simulink model "cdma2000_phlayer"  (Simulink 6.0)
settings: Solver=FixedStepDiscrete  SolverMode=SingleTasking  StartTime=0.0  StopTime=1  RelTol=1e-3
PreLoadFcn:
  | % Create interleaver table
  | % By default, numSampInt is set to 768 and radConfig to 3
  | interTable = cdma2000_inttable(768, 3);
undefined symbols (not defined in the file or in its folder): figposition, Fs, Non, slcm, TD
libraries: cdma2000_lib x8, commsink2 x5, commsequence2 x3, dspsigops x3, dspsnks4 x2, commblkintrlv2 x2, commcrc2 x2, commcnvcod2 x2, commrandsrc2 x1, commutil2 x1, dspsrcs4 x1
CloseFcn:
  | % Clear interleaver Table
  | clear interTable;
  | % Clear error string
  | clear eStr;
  | % Clear signal logging
  | clear cdma2000SigsOut;
settings Model: Creator=arodrigu  LastModifiedBy=arodrigu  ProdHWDeviceType=Specified
settings DataIOCC: LimitDataPoints=off  SaveOutput=off  SaveTime=off  SignalLoggingName=cdma2000SigsOut
settings OptimizationCC: BooleanDataType=off  InlineInvariantSignals=off
settings DebuggingCC: CheckExecutionContextPreStartOutputMsg=on  CheckExecutionContextRuntimeOutputMsg=on  SolverPrmCheckMsg=none  InheritedTsInSrcMsg=none
settings HardwareCC: ProdHWDeviceType=Specified
settings ModelReferenceCC: UpdateModelReferenceTargets=IfOutOfDate
settings CodeAppCC: MangleLength=5

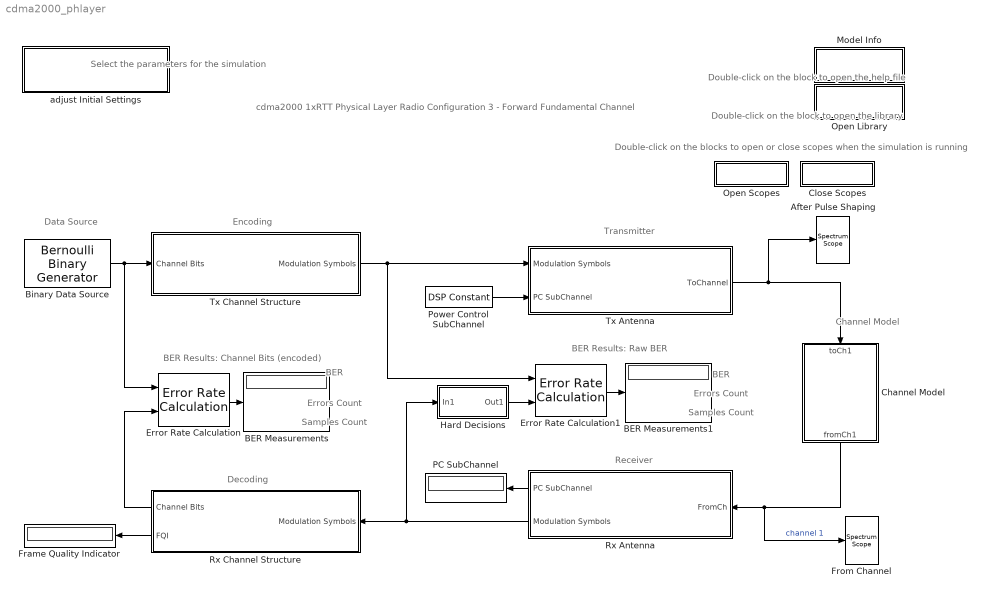
== system cdma2000_phlayer ==
  note: cdma2000 1xRTT Physical Layer
      | Radio Configuration 3 - Forward Fundamental Channel
  note: Double-click on the block
      | to open the help file
  note: BER
  note: Errors Count
  note: Samples Count
  note: BER
  note: Errors Count
  note: Samples Count
  note: Transmitter
  note: Receiver
  note: Channel
      | Model
  note: Encoding
  note: Decoding
  note: Select the parameters
      | for the simulation
  note: BER Results: Raw BER
  note: BER Results: Channel Bits (encoded)
  note: Double-click on the block
      | to open the library
  note: Double-click on the blocks to open or close scopes
      | when the simulation is running
  note: Data Source
  After Pulse Shaping : dspsnks4/Spectrum Scope  ScopeProperties=off  Domain=Frequency  HorizSpan=1  UseBuffer=on  BufferSize=256  Overlap=0  inpFftLenInherit=off  FFTlength=128  numAvg=20  DisplayProperties=on  AxisGrid=on  Memory=off  FrameNumber=off  AxisLegend=off  AxisZoom=off  OpenScopeAtSimStart=off  OpenScopeImmediately=off  FigPos="figposition([7    12    39    27])"  AxisProperties=off  XUnits=Hertz  XRange=[-Fs/2...Fs/2]  InheritXIncr=on  XIncr=1.0  XLabel=Samples  YUnits=dB  YLabel=Magnitude, dB  LineProperties=off  LineColors=[1 0 0]
      settings: YMin=-50.9192306956859  YMax=14.9570095672604
  BER Measurements : Display
  BER Measurements1 : Display
  Binary Data Source : commrandsrc2/Bernoulli Binary Generator  P=0.5  seed=1234  Ts=20e-3*1/172  frameBased=on  sampPerFrame=172  orient=off
      settings: AttributesFormatString=Samples per Frame = %<sampPerFrame>\nSample Time = %<Ts>
  Channel Model : Subsystem  Orientation=down  PropExecContextAcrossSSBoundary=on
      mask Display: disp('Channel\nModels');
  Close Scopes : Subsystem  PropExecContextAcrossSSBoundary=on
      settings: OpenFcn=|
      | str1 = 'Rx Antenna';
      | str2 = 'From Channel';
      | str3 = 'After Rake';
      | str5 = 'After Derotation';                                        str6 = 'After Pulse Shaping';
      | str7 = 'From Channel';
      | 
      | 
      | sdspfscope2([],[],[],'ScopeUpdate',[bdroot '/' str1 '/' str2 ],'CloseFig');
      | sdspfscope2([],[],[],'ScopeUpdate',[bdroot '/' str1 '/' str3 ],'CloseFig');
      | sdspfscope2([],[],[],'ScopeUpdate',[bdroot '/' str1 '/' str5 ],'CloseFig');
      | sdspfscope2([],[],[],'ScopeUpdate',[bdroot '/' str6],'CloseFig');
      |  sdspfscope2([],[],[],'ScopeUpdate',[bdroot '/' str7],'CloseFig');
      mask Display: disp('Close Scopes');
  Error Rate Calculation : commsink2/Error Rate Calculation  N=2*172  st_delay=0  cp_mode=Entire frame  subframe=[]  PMode=Port  WsName=ErrorVec  RsMode2=off  stop=off  numErr=100  maxBits=1e6
      settings: AttributesFormatString=Received Delay = %<N>
  Error Rate Calculation1 : commsink2/Error Rate Calculation  N=2*768  st_delay=0  cp_mode=Entire frame  subframe=[]  PMode=Port  WsName=ErrorVec  RsMode2=off  stop=off  numErr=100  maxBits=1e6
      settings: AttributesFormatString=Received Delay = %<N>
  Frame Quality Indicator : Display
  From Channel : dspsnks4/Spectrum Scope  ScopeProperties=off  Domain=Frequency  HorizSpan=1  UseBuffer=on  BufferSize=512  Overlap=0  inpFftLenInherit=off  FFTlength=128  numAvg=2  DisplayProperties=on  AxisGrid=on  Memory=off  FrameNumber=off  AxisLegend=off  AxisZoom=off  OpenScopeAtSimStart=off  OpenScopeImmediately=off  FigPos="figposition([49    12    39    27])"  AxisProperties=off  XUnits=Hertz  XRange=[-Fs/2...Fs/2]  InheritXIncr=on  XIncr=1.0  XLabel=Samples  YUnits=dB  YLabel=Magnitude, dB  LineProperties=off  LineColors=[1 0 0]
      settings: YMin=-25.3833693734741  YMax=21.0980719822277
  Hard Decisions : Subsystem  PropExecContextAcrossSSBoundary=on
      mask Display: disp('Hard\nDecisions');
  Model Info : Subsystem  LoadFcn=slcm LoadBlock;  InitFcn=slcm('UpdateAllCMBlocksInThisModelInit')  PropExecContextAcrossSSBoundary=on  mask(CMBlock){InitialSaveTempField=, InitialBlockCM=None, BlockCM=None, Frame=on, SaveTempField=, DisplayStringWithTags=Info, MaskDisplayString=Info, HorizontalTextAlignment=Center, LeftAlignmentValue=0.5, SourceBlockDiagram=cdma2000_phlayer, TagMaxNumber=20, CMTag1=, CMTag2=, CMTag3=, CMTag4=, CMTag5=, CMTag6=, CMTag7=, CMTag8=, CMTag9=, CMTag10=, CMTag11=, CMTag12=, CMTag13=, CMTag14=, CMTag15=, CMTag16=, CMTag17=, CMTag18=, CMTag19=, CMTag20=}
      mask help: This block allows revision control information to be displayed within the model.
      settings: CopyFcn=slcm CopyBlock;  DeleteFcn=slcm Cancel;  PostSaveFcn=slcm('UpdateAllCMBlocksInThisModel')  NameChangeFcn=slcm Rename;  OpenFcn=commdemohelp;
      mask Display: text(str2num(LeftAlignmentValue), 0.5, MaskDisplayString, 'HorizontalAlignment', HorizontalTextAlignment)
  Open Library : Subsystem  PropExecContextAcrossSSBoundary=on
      settings: OpenFcn=open('cdma2000_lib.mdl');
      mask Display: disp('cdma2000\nLibrary')
  Open Scopes : Subsystem  PropExecContextAcrossSSBoundary=on
      settings: OpenFcn=|
      | str1 = 'Rx Antenna';
      | str2 = 'From Channel';
      | str3 = 'After Rake';
      | str5 = 'After Derotation';
      | str6 = 'After Pulse Shaping';
      | str7 = 'From Channel';
      | 
      | sdspfscope2([],[],[],'ScopeUpdate',[bdroot '/' str1 '/' str2 ],'OpenFig');
      | sdspfscope2([],[],[],'ScopeUpdate',[bdroot '/' str1 '/' str3 ],'OpenFig');
      | sdspfscope2([],[],[],'ScopeUpdate',[bdroot '/' str1 '/' str5 ],'OpenFig');
      | sdspfscope2([],[],[],'ScopeUpdate',[bdroot '/' str6],'OpenFig');
      |  sdspfscope2([],[],[],'ScopeUpdate',[bdroot '/' str7],'OpenFig');
      mask Display: disp('Open Scopes');
  PC SubChannel : Display
  Power Control SubChannel : dspsrcs4/DSP Constant  Value=1  SampleMode=Discrete  discreteOutput=Frame-based  continuousOutput=Sample-based  sampTime=20e-3/16  framePeriod=20e-3/16  dataType=Inherit from 'Constant value'  isSigned=on  wordLen=16  udDataType=sfix(16)  fracBitsMode=Best precision  numFracBits=15  InterpretAs1D=off  Ts=20e-3/16  FramebasedOutput=on
      settings: AttributesFormatString=\n\n\n\n
  Rx Antenna : Subsystem  Orientation=left  PropExecContextAcrossSSBoundary=on
  Rx Channel Structure : Subsystem  Orientation=left  PropExecContextAcrossSSBoundary=on
  Tx Antenna : Subsystem  PropExecContextAcrossSSBoundary=on
  Tx Channel Structure : Subsystem  PropExecContextAcrossSSBoundary=on
      mask Display:
      | port_label('output',1,'Modulation Symbols');
      | port_label('input',1,'Channel Bits');
  adjust Initial Settings : Subsystem  PropExecContextAcrossSSBoundary=on  mask(cdma2000 Initial Settings){chType=Forward Fundamental, radConfig=Radio Configuration 3, dataRates=9.6 Kbps, nFrameMask=1, longCScrMask=On, gateRateMask=1/4, trChCode=23, pnOffset=1, qof_idx=2, TxDivMode=Non-TD, chMode1=Multipath Fading Channel, EcN0=10, dopplerFreq=486, delayVector=[0 260e-9 521e-9 781e-9], gainVector=[0 -3 -6 -9]}
      mask prompts: chType "Channel Type"; radConfig "Radio Configuration"; dataRates "Data Rates:"; nFrameMask "Length of frame in multiples of 20 ms (n):"; longCScrMask "Long Code Scrambling:"; gateRateMask "Power Control SubChannel Insertion Rate:"; trChCode "Forward Traffic Channel Spreading Code Index:"; pnOffset "Forward Traffic Channel PN Offset:"; qof_idx "Quasi-orthogonal function index for F-DTCH:"; TxDivMode "Transmit Diversity Mode:"; chMode1 "Channel Model:"; EcN0 "EcN0 (in dB):"; dopplerFreq "Maximum Doppler Frequency shift (in Hz):"; delayVector "Multipath Profile - Delay Vector (s):"; gainVector "Multipath Profile - Gain Vector (dB):"
      mask help:
      | Select the parameters for the cdma200 application example.
      |
      | Some options have been disabled because they are not supported in this example. These options are intentionally displayed to exemplify possible ways to expand the model.
      mask init:
      | eStr = cdma2000_initmask(gcb, 'init');
      | if(~isempty(eStr.emsg))
      | errordlg(eStr.emsg);
      | end
      settings: AttributesFormatString=%<chType>\n%<radConfig>\n%<dataRates>\n%<txDivMode>\n%<chMode1>\n
      mask Help: eval('commdemohelp;');
      mask StyleString: popup(Forward Fundamental),popup(Radio Configuration 3),popup(1.5 Kbps|2.7 Kbps|4.8 Kbps|9.6 Kbps),popup(1|2|4),popup(On|Off),popup(Non Power Control|1|1/2|1/4),edit,edit,popup(0|1|2|3),popup(Non-TD),popup(No Channel|AWGN Channel|Multipath Fading Channel),edit,edit,edit,edit
      mask CallbackString: ||cdma2000_initmask(gcb,'cbDataRates');|cdma2000_initmask(gcb,'cbNFrameMask');|cdma2000_initmask(gcb,'cbLongCScrMask');|cdma2000_initmask(gcb,'cbGateRateMask');|cdma2000_initmask(gcb,'cbTrChCode');|cdma2000_initmask(gcb,'cbPnOffset');|cdma2000_initmask(gcb,'cbQof_idx');|cdma2000_initmask(gcb,'cbTxDivMode');|cdma2000_initmask(gcb,'cbChMode1');||||
      mask Display: disp('cdma2000:\nInitial Settings');
  wires:
  Binary Data Source/1 -> Tx Channel Structure/1(Channel Bits), Error Rate Calculation/1
  Error Rate Calculation/1 -> BER Measurements/1
  Error Rate Calculation1/1 -> BER Measurements1/1
  Tx Antenna/1(ToChannel) -> Channel Model/1(toCh1), After Pulse Shaping/1
  Channel Model/1(fromCh1) -> Rx Antenna/1(FromCh), From Channel/1  "channel 1"
  Tx Channel Structure/1(Modulation Symbols) -> Error Rate Calculation1/1, Tx Antenna/1(Modulation Symbols)
  Rx Channel Structure/1(Channel Bits) -> Error Rate Calculation/2
  Rx Channel Structure/2(FQI) -> Frame Quality Indicator/1
  Power Control SubChannel/1 -> Tx Antenna/2(PC SubChannel)
  Rx Antenna/1(PC SubChannel) -> PC SubChannel/1
  Rx Antenna/2(Modulation Symbols) -> Rx Channel Structure/1(Modulation Symbols), Hard Decisions/1(In1)
  Hard Decisions/1(Out1) -> Error Rate Calculation1/2

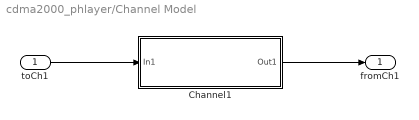
== system cdma2000_phlayer/Channel Model ==
  toCh1 : Inport  LatchInput=off
  Channel1 : Subsystem  BlockChoice=Multipath Fading Channel  PropExecContextAcrossSSBoundary=on
      link override AWGN Channel: EsNodB=10
      link override Multipath Fading Channel: EcN0=10  dopplerFreq=486  delayVector="[0    2.6e-007   5.21e-007   7.81e-007]"  gainVector=[0 -3 -6 -9]
      link override Multipath Fading Channel/AWGN Channel: EsNodB=EcN0
      link override Multipath Fading Channel/Multipath Rayleigh Fading Channel: Fd=dopplerFreq  delayVec=delayVector  gainVecdB=gainVector
      settings: AttributesFormatString=%<BlockChoice>  MemberBlocks=AWGN Channel,Multipath Fading Channel,No Channel
      settings: TemplateBlock=|
      | cdma2000_lib/cdma2000 Channel Models/Configurable
      | Subsystem
  fromCh1 : Outport
  wires:
  toCh1/1 -> Channel1/1(In1)
  Channel1/1(Out1) -> fromCh1/1

== system cdma2000_phlayer/Close Scopes ==
  note: This subsystem is intentionally left empty

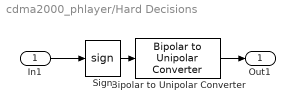
== system cdma2000_phlayer/Hard Decisions ==
  In1 : Inport  LatchInput=off
  Bipolar to Unipolar Converter : commutil2/Bipolar to Unipolar Converter  M=2  polarity=Negative
  Sign : Signum
  Out1 : Outport
  wires:
  Sign/1 -> Bipolar to Unipolar Converter/1
  Bipolar to Unipolar Converter/1 -> Out1/1
  In1/1 -> Sign/1

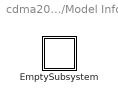
== system cdma2000_phlayer/Model Info ==
  EmptySubsystem : Subsystem  PropExecContextAcrossSSBoundary=on

== system cdma2000_phlayer/Open Library ==
  note: This subsystem is intentionally left empty

== system cdma2000_phlayer/Open Scopes ==
  note: This subsystem is intentionally left empty

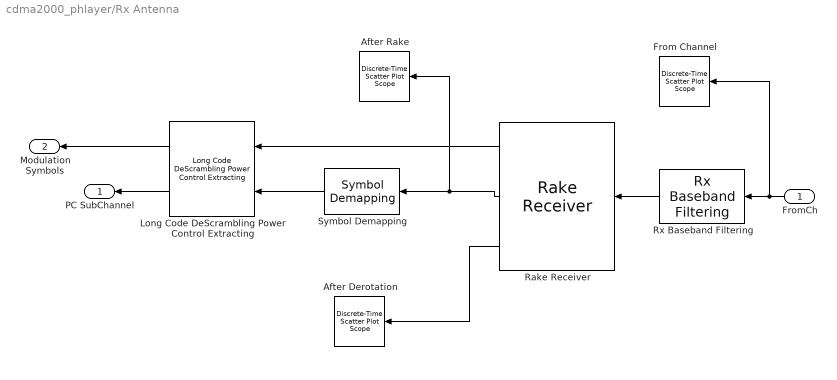
== system cdma2000_phlayer/Rx Antenna ==
  FromCh : Inport  Orientation=left  LatchInput=off
  After Derotation : commsink2/Discrete-Time Scatter Plot Scope  Tag=ScatterPlot  Orientation=left  sampPerSymb=1  offsetEye=0  numTraces=100  numNewFrames=20  LineMarkers=.  LineColors=b  fading=on  render=off  AxisGrid=on  xMin=-3.22434444007457  xMax=3.46614847196624  yMin=-3.31792338934159  yMax=3.37256952269922  inphaseLabel=After Derotation  quadratureLabel=""  openScopeAtSimStart=off  FrameNumber=off  FigPos="figposition([36    51    30    40])"  figTitle=.  numLinesMax=50  block_type_=scatter
  After Rake : commsink2/Discrete-Time Scatter Plot Scope  Tag=ScatterPlot  Orientation=left  sampPerSymb=1  offsetEye=0  numTraces=100  numNewFrames=40  LineMarkers=.  LineColors=[1 0 1]  fading=on  render=off  AxisGrid=on  xMin=-2.7  xMax=2.7  yMin=-2.7  yMax=2.7  inphaseLabel=After Rake Receiver  quadratureLabel=""  openScopeAtSimStart=off  FrameNumber=off  FigPos="figposition([68    51    30    40])"  figTitle=.  numLinesMax=50  block_type_=scatter
  From Channel : commsink2/Discrete-Time Scatter Plot Scope  Tag=ScatterPlot  Orientation=left  sampPerSymb=1  offsetEye=0  numTraces=3000  numNewFrames=2000  LineMarkers=.  LineColors=[1 0 1]  fading=on  render=off  AxisGrid=on  xMin=-2.7  xMax=2.7  yMin=-2.7  yMax=2.7  inphaseLabel=From Channel  quadratureLabel=""  openScopeAtSimStart=off  FrameNumber=off  FigPos="figposition([4    51    30    40])"  figTitle=.  numLinesMax=50  block_type_=scatter
  Long Code DeScrambling Power Control Extracting : cdma2000_lib/cdma2000 Receiver/Long Code DeScrambling Power Control Extracting  Orientation=left  radConfig=Radio Configuration 3  numSamp=768  nFrameMask=1  longCScrMask=On  gateRateMask=1/4  TxDivMode=Non-TD  plcMask="[1 1 0 0 0 1  1  0  0  1  1  0  1  0  1  1  1  1  0  1  1  0  0  1  0  1  1  1  0  0  1  0  1  0  1  1  1  1  0  1  1  0]"
  Rake Receiver : cdma2000_lib/cdma2000 Receiver/Rake Receiver  Orientation=left  walshLength=64  trChCode=23  pnOffset=1  qof_idx=2  numTapsChEst=11  numTapsRRC=48  overSampling=4  fingerEnables="[1  1  1  1]"  fingerPhases="[0  1  3  4]"
  Rx Baseband Filtering : cdma2000_lib/cdma2000 Receiver/Rx Baseband Filtering  Orientation=left
  Symbol Demapping : cdma2000_lib/cdma2000 Receiver/Symbol Demapping  Orientation=left
  PC SubChannel : Outport  Orientation=left
  Modulation Symbols : Outport  Orientation=left  Port=2
  wires:
  Rake Receiver/2 -> Symbol Demapping/1, After Rake/1
  Rake Receiver/1 -> Long Code DeScrambling Power Control Extracting/1
  Rx Baseband Filtering/1 -> Rake Receiver/1
  Long Code DeScrambling Power Control Extracting/1 -> Modulation Symbols/1
  FromCh/1 -> Rx Baseband Filtering/1, From Channel/1
  Long Code DeScrambling Power Control Extracting/2 -> PC SubChannel/1
  Rake Receiver/3 -> After Derotation/1
  Symbol Demapping/1 -> Long Code DeScrambling Power Control Extracting/2

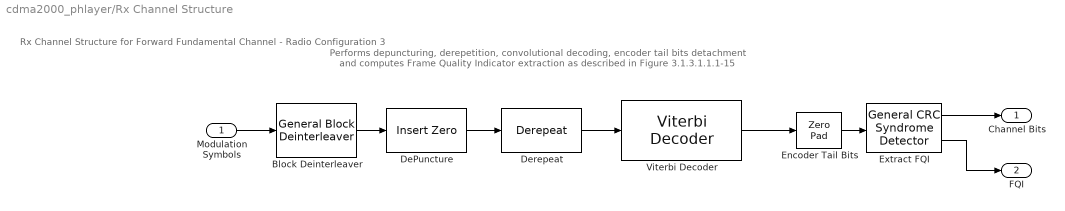
== system cdma2000_phlayer/Rx Channel Structure ==
  note: Rx Channel Structure for
      | Forward Fundamental Channel - Radio Configuration 3
  note: Performs depuncturing, derepetition, convolutional decoding, encoder tail bits detachment and computes
      | Frame Quality Indicator extraction as described in Figure 3.1.3.1.1.1-15
  Modulation Symbols : Inport  LatchInput=off
  Block Deinterleaver : commblkintrlv2/General Block Deinterleaver  elements=interTable
  DePuncture : commsequence2/Insert Zero  insertZeroVector=[1]
  Derepeat : commsequence2/Derepeat  N=1  ic=0  mode=Maintain input frame rate
  Encoder Tail Bits : dspsigops/Zero Pad  padSigAt=End  zpadAlong=Columns  padNumOutRowsSpecMethod=User-specified  numOutRows=172 + 12  padNumOutColsSpecMethod=User-specified  numOutCols=1  trunc_flag=None
  Extract FQI : commcrc2/General CRC Syndrome Detector  genPoly=[12 11 10 9 8 4 1 0]  iniStates=[1]  numChecksums=1
  Viterbi Decoder : commcnvcod2/Viterbi Decoder  trellis=poly2trellis(9, [765 671 513 473])  dectype=Unquantized  nsdecb=4  tbdepth=30  opmode=Truncated  reset=off
  Channel Bits : Outport
  FQI : Outport  Port=2
  wires:
  Block Deinterleaver/1 -> DePuncture/1
  Extract FQI/1 -> Channel Bits/1
  Extract FQI/2 -> FQI/1
  Encoder Tail Bits/1 -> Extract FQI/1
  Modulation Symbols/1 -> Block Deinterleaver/1
  Viterbi Decoder/1 -> Encoder Tail Bits/1
  Derepeat/1 -> Viterbi Decoder/1
  DePuncture/1 -> Derepeat/1

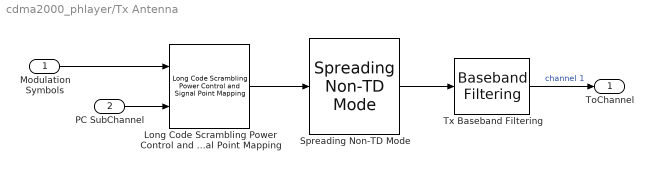
== system cdma2000_phlayer/Tx Antenna ==
  Modulation Symbols : Inport  LatchInput=off
  PC SubChannel : Inport  Port=2  LatchInput=off
  Long Code Scrambling Power Control and Signal Point Mapping : cdma2000_lib/cdma2000 Transmitter/Long Code Scrambling Power Control and Signal Point Mapping  radConfig=Radio Configuration 3  numSamp=768  nFrameMask=1  longCScrMask=On  gateRateMask=1/4  TxDivMode=Non-TD  plcMask="[1 1 0 0 0 1  1  0  0  1  1  0  1  0  1  1  1  1  0  1  1  0  0  1  0  1  1  1  0  0  1  0  1  0  1  1  1  1  0  1  1  0]"
  Spreading Non-TD Mode : cdma2000_lib/cdma2000 Transmitter/Spreading Non-TD Mode  walshLength=64  trChCode=23  qof_idx=2  pnOffset=1
  Tx Baseband Filtering : cdma2000_lib/cdma2000 Transmitter/Baseband Filtering
  ToChannel : Outport
  wires:
  PC SubChannel/1 -> Long Code Scrambling Power Control and Signal Point Mapping/2
  Long Code Scrambling Power Control and Signal Point Mapping/1 -> Spreading Non-TD Mode/1
  Spreading Non-TD Mode/1 -> Tx Baseband Filtering/1
  Modulation Symbols/1 -> Long Code Scrambling Power Control and Signal Point Mapping/1
  Tx Baseband Filtering/1 -> ToChannel/1  "channel 1"

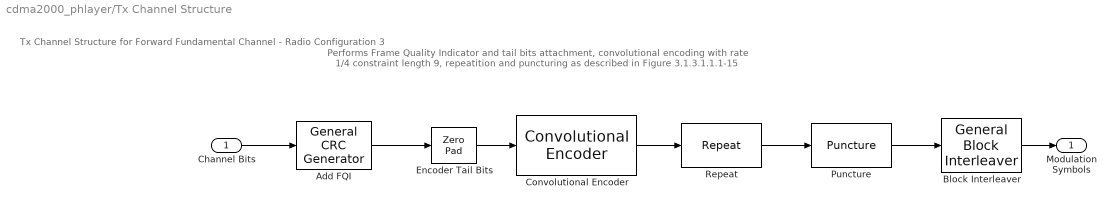
== system cdma2000_phlayer/Tx Channel Structure ==
  note: Tx Channel Structure for
      | Forward Fundamental Channel - Radio Configuration 3
  note: Performs Frame Quality Indicator and tail bits attachment, convolutional encoding with rate 1/4 constraint length 9,
      | repeatition and puncturing as described in Figure 3.1.3.1.1.1-15
  Channel Bits : Inport  LatchInput=off
  Add FQI : commcrc2/General CRC Generator  genPoly=[12 11 10 9 8 4 1 0]  iniStates=[1]  numChecksums=1
  Block Interleaver : commblkintrlv2/General Block Interleaver  elements=interTable
  Convolutional Encoder : commcnvcod2/Convolutional Encoder  trellis=poly2trellis(9, [765 671 513 473])  reset=On each frame
  Encoder Tail Bits : dspsigops/Zero Pad  padSigAt=End  zpadAlong=Columns  padNumOutRowsSpecMethod=User-specified  numOutRows=172 + 12 + 8  padNumOutColsSpecMethod=User-specified  numOutCols=1  trunc_flag=None
  Puncture : commsequence2/Puncture  punctureVector=[1]
  Repeat : dspsigops/Repeat  N=1  ic=0  mode=Maintain input frame rate
  Modulation Symbols : Outport
  wires:
  Block Interleaver/1 -> Modulation Symbols/1
  Channel Bits/1 -> Add FQI/1
  Add FQI/1 -> Encoder Tail Bits/1
  Encoder Tail Bits/1 -> Convolutional Encoder/1
  Convolutional Encoder/1 -> Repeat/1
  Repeat/1 -> Puncture/1
  Puncture/1 -> Block Interleaver/1

== system cdma2000_phlayer/adjust Initial Settings ==
  note: This subsystem is intentionally left empty

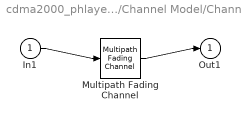
== system cdma2000_phlayer/Channel Model/Channel1 ==
  In1 : Inport  LatchInput=off
  Multipath Fading Channel : cdma2000_lib/cdma2000 Channel Models/Multipath Fading Channel  EcN0=10  dopplerFreq=486  delayVector="[0    2.6e-007   5.21e-007   7.81e-007]"  gainVector=[0 -3 -6 -9]
  Out1 : Outport
  wires:
  In1/1 -> Multipath Fading Channel/1
  Multipath Fading Channel/1 -> Out1/1

== system cdma2000_phlayer/Model Info/EmptySubsystem ==
